simulink model "WT_PUBLICATION_MODEL"  (R2025a)
settings: Solver=ode4  StartTime=0.0  StopTime=11  FixedStep=0.1  RelTol=1e-3
libraries: simulink x1
settings Model: Creator=hero  LastModifiedBy=hero

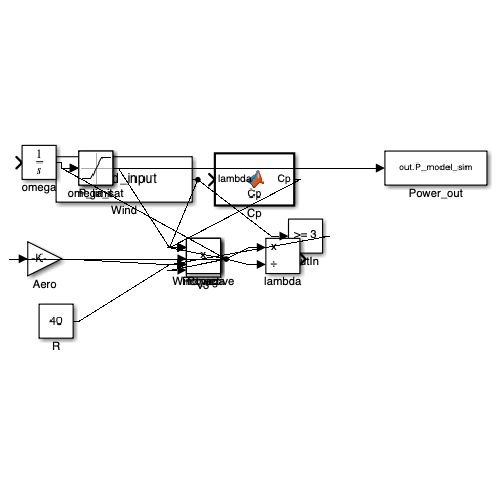
[thumbnail: Simulink's stored preview of the top-level diagram]
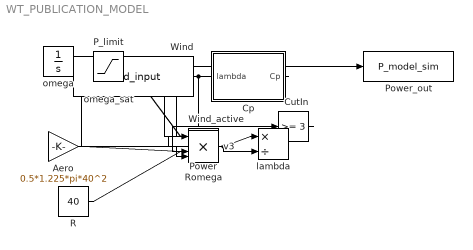
== system WT_PUBLICATION_MODEL ==
  Aero : Gain  Gain=0.5*1.225*pi*40^2
  Cp : MATLAB Function  TreatAsAtomicUnit=on
  CutIn : simulink/Logic and Bit Operations/Compare To Constant  relop=>=  const=3  OutDataTypeStr=boolean
  P_limit : Saturate  UpperLimit=652.7945  LowerLimit=0
  Power : Product
  Power_out : ToWorkspace  VariableName=P_model_sim  SampleTime=-1
  R : Constant  Value=40
  Romega : Product
  Wind : FromWorkspace  VariableName=wind_input
  Wind_active : Product
  lambda : Product  Inputs=*/
  omega : Integrator  InitialCondition=10
  omega_sat : Saturate  UpperLimit=100  LowerLimit=0.5
  v3 : Product  Inputs=3
  wires:
  Wind/1 -> CutIn/1, Wind_active/1
  CutIn/1 -> Wind_active/2
  omega/1 -> omega_sat/1
  omega_sat/1 -> Romega/1
  R/1 -> Romega/2
  Romega/1 -> lambda/1
  Wind_active/1 -> lambda/2, v3/1, v3/2, v3/3
  v3/1 -> Aero/1
  Aero/1 -> Power/2
  Cp/1(Cp) -> Power/1
  Power/1 -> P_limit/1
  P_limit/1 -> Power_out/1

== matlab function WT_PUBLICATION_MODEL/Cp ==
  data: lambda input; Cp output
function Cp = Cp(lambda)
lambda = max(lambda,0.1);
lambda = min(lambda,12);
% Smooth peak around lambda_opt
Cp = 0.48 * exp(-((lambda-8).^2)/10);
end
